simulink model "Q7"  (R2020a)
settings: Solver=VariableStepAuto  StartTime=0.0  StopTime=50.0  RelTol=1e-3
settings Model: Creator=emami  LastModifiedBy=emami

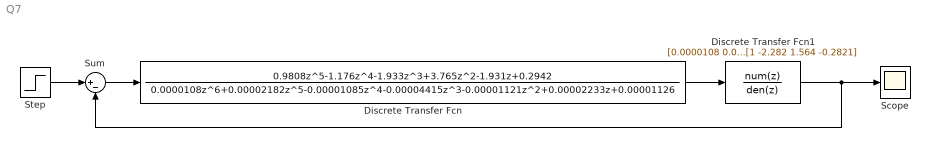
== system Q7 ==
  Discrete Transfer Fcn : DiscreteTransferFcn  Numerator=[0.9808 -1.176 -1.933 3.765 -1.931 0.2942]  Denominator=[0.0000108 0.00002182 -0.00001085 -0.00004415 -0.00001121 0.00002233 0.00001126]
  Discrete Transfer Fcn1 : DiscreteTransferFcn  Numerator=[0.0000108 0.00003241 0.00003241 0.0000108]  Denominator=[1 -2.282 1.564 -0.2821]
  Scope : Scope
  Step : Step  SampleTime=0
  Sum : Sum  Inputs=|+-
  wires:
  Step/1 -> Sum/1
  Sum/1 -> Discrete Transfer Fcn/1
  Discrete Transfer Fcn/1 -> Discrete Transfer Fcn1/1
  Discrete Transfer Fcn1/1 -> Scope/1, Sum/2
